simulink model "test_connectivity_ns3"  (R2024b)
settings: Solver=FixedStepAuto  StartTime=0.0  StopTime=100.0  FixedStep=0.0001  RelTol=1e-3
undefined symbols (not defined in the file or in its folder): f
libraries: slrealtimeiplib x2, instrumentlib x2
settings Model: Creator=hnh21  LastModifiedBy=hnh21

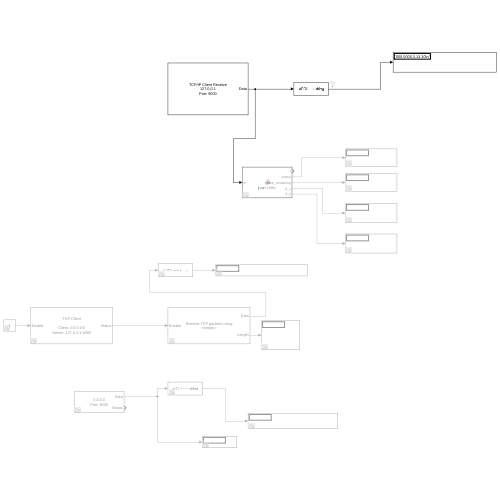
[thumbnail: Simulink's stored preview of the top-level diagram]
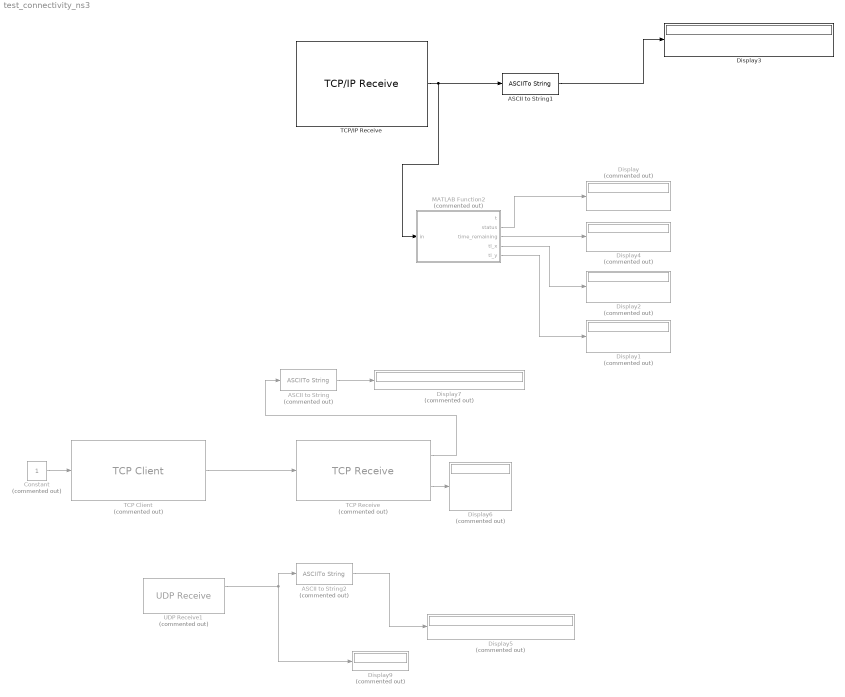
== system test_connectivity_ns3 ==
  ASCII to String : ASCIIToString  Commented=on
  ASCII to String1 : ASCIIToString
  ASCII to String2 : ASCIIToString  Commented=on
  Constant : Constant  Commented=on
  Display{,1..2,4..7,9} (8 alike) : Display  Commented=on
  Display3 : Display
  MATLAB Function2 : MATLAB Function  Commented=on  TreatAsAtomicUnit=on
  TCP Client : slrealtimeiplib/TCP Client  Priority=-1  Commented=on  useHostTargetConn=off  remoteAddress=127.0.0.1  remotePort=9000
  TCP Receive : slrealtimeiplib/TCP Receive  Commented=on  socketAddPortVal=<empty>  rcvWidth=38  sampleTime=0.0001
  TCP/IP Receive : instrumentlib/TCP//IP Receive  Host=127.0.0.1  Port=9000  DataSize=17  DataType=uint8  ASCIIFormatting=%f  Terminator=LF  CustomTerminator=10  ByteOrder=big-endian  EnableBlockingMode=on  Timeout=0.5  SampleTime=0.001  SimulateUsing=Interpreted execution
  UDP Receive1 : instrumentlib/UDP Receive  Commented=on  LocalAddress=0.0.0.0  LocalPort=9000  EnablePortSharing=off  Host=127.0.0.1  Port=9000  GetLatestData=off  DataSize=38  DataType=uint8  ASCIIFormatting=%f,  Terminator=LF  CustomTerminator=10  ByteOrder=big-endian  EnableBlockingMode=off  Timeout=1  SampleTime=0.0001  SimulateUsing=Interpreted execution
  wires:
  TCP/IP Receive/1 -> MATLAB Function2/1(in), ASCII to String1/1
  ASCII to String1/1 -> Display3/1
  MATLAB Function2/5(tl_y) -> Display1/1
  MATLAB Function2/4(tl_x) -> Display2/1
  MATLAB Function2/2(status) -> Display/1
  MATLAB Function2/3(time_remaining) -> Display4/1
  TCP Client/1 -> TCP Receive/1
  TCP Receive/1 -> ASCII to String/1
  TCP Receive/2 -> Display6/1
  Constant/1 -> TCP Client/1
  ASCII to String/1 -> Display7/1
  UDP Receive1/1 -> Display9/1, ASCII to String2/1
  ASCII to String2/1 -> Display5/1

== matlab function test_connectivity_ns3/MATLAB Function2 ==
  data: in input; t output; status output; time_remaining output; tl_x output; tl_y output
function [t, status, time_remaining, tl_x, tl_y] = parseMsg(in)
%#codegen

% Define max buffer size
MAX_LEN = 256;

% Persistent buffer and index
persistent buffer idx

if isempty(buffer)
    buffer = zeros(1, MAX_LEN, 'uint8');  % uint8 buffer
    idx = 0;
end

% Initialize outputs
t = 0.0;
status = 0;
time_remaining = 0.0;
tl_x = 0.0;
tl_y = 0.0;

% Process input
for i = 1:length(in)
    b = uint8(in(i));

    if idx < MAX_LEN
        idx = idx + 1;
        buffer(idx) = b;
    end

    if b == 10  % newline
        line = char(buffer(1:idx-1));  % remove newline
        tokens = sscanf(line, '%f,%d,%f,%f,%f');  % read first 5 fields
        if numel(tokens) >= 5
            t = tokens(1);
            status = tokens(2);
            time_remaining = tokens(3);
            tl_x = tokens(4);
            tl_y = tokens(5);
        end
        idx = 0;  % reset buffer
    end
end
